simulink model "2025.1.21.methods"  (R2023a)
settings: Solver=ode4  StartTime=0.0  StopTime=40  FixedStep=dt  RelTol=1e-3
values from neighbouring files (symbols this model uses):
  AgN = Ag    [Copy_of_New_Ns.m]    (also in 旧数值子结构.m = zeros(ndof,1))
  C_phys_5dof = C    [旧静力凝聚.m]
  CNrt = CRrt    [Copy_of_New_Ns.m]    (also in 旧数值子结构.m)
  FN = zeros(15,1)    [Copy_of_New_Ns.m]    (also in 旧数值子结构.m = zeros(ndof,1))
  K_phys_5dof = K    [旧静力凝聚.m]
  KNbar_inv = inv(KNbar)    [Copy_of_New_Ns.m]    (also in 旧数值子结构.m)
  Koo = K(3:end,3:end)    [旧静力凝聚.m]
  Kot = K(3:end,1:2)    [旧静力凝聚.m]
  lN = l    [Copy_of_New_Ns.m]    (also in 旧数值子结构.m = zeros(ndof,1))
  M_phys_5dof = M    [旧静力凝聚.m]
  MNrt = diag([M1 1e-5 M6 M3 M2 M4 1e-5 M6 M3 M2 M1 M2 M3 M3 M2])    [Copy_of_New_Ns.m]    (also in 旧数值子结构.m = csvread("FE_Model/REF_SAP2000_Model/M_matrix.csv"))
  RNbar = zeros(15,1)    [Copy_of_New_Ns.m]    (also in 旧数值子结构.m = zeros(ndof,1))
undefined symbols (not defined in the file or in its folder): a0, a1, a2, a3, a4, a5, a6, a7, A_cplant, alpha1, alpha2, B_cplant, C_cplant, D_cplant, Dd_ss, delay, Ds_ss, dt, dv1, dv2, EQ_intensity, EQ_sw, Gnd_ss, Gns_ss, Hs1, Hs2, k3, k4, k6, K_lqr, KE, Mren, Muu, Phi_u2, Seed_snr
libraries: simulink x2, slpidlib x2, sldrtlib x1
(part 1 of 2)
settings Model: Creator=icu327  LastModifiedBy=liangyu
settings SolverCC: AlgebraicLoopSolver=TrustRegion
settings DataIOCC: SaveFormat=Array  ReturnWorkspaceOutputs=off
settings DebuggingCC: UnconnectedInputMsg=warning  UnconnectedOutputMsg=warning  UnconnectedLineMsg=warning  ArithmeticOperatorsInVariantConditions=warning
settings HardwareCC: ProdBitPerLong=64  ProdHWDeviceType=Intel->x86-64 (Linux 64)
settings ModelReferenceCC: EnableRefExpFcnMdlSchedulingChecks=on
settings SFSimCC: CustomCodeUndefinedFunction=UseInterfaceOnly
settings RTWCC: Description=Simulink Desktop Real-Time  SystemTargetFile=sldrt.tlc  TemplateMakefile=sldrt.tmf  RTWCompilerOptimization=on
settings CodeAppCC: MaxIdLength=95  StateflowObjectComments=on
settings SimulinkDesktopRealTimeCC: TargetLibSuffix=_sldrt.a  TargetPreCompLibLocation=C:\Program Files\MATLAB\R2023a\toolbox\sldrt\lib\win64

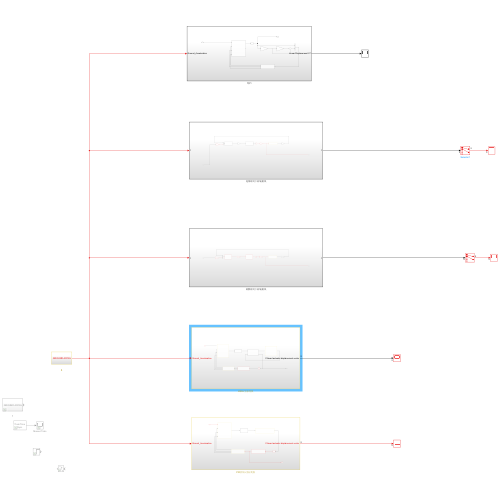
[thumbnail: Simulink's stored preview of the top-level diagram]
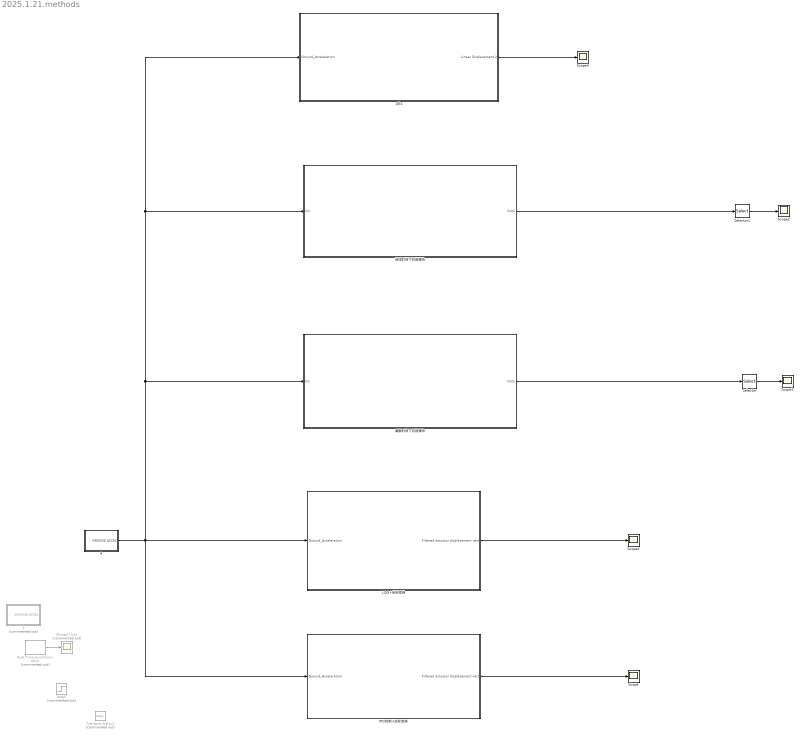
== system 2025.1.21.methods ==
  " 1" : Subsystem  Commented=on
  " 4" : Subsystem
  1阶1 : Subsystem
  LQG+坐标变换 : Subsystem
  Missed Ticks : Scope  Commented=on
  PID控制+坐标变换 : Subsystem
  Real-Time Synchronization : sldrtlib/Real-Time Synchronization  Commented=on  SampleTime=dt  MaxMissedTicks=10000  ShowMissedTicks=on  YieldWhenWaiting=off
  Scope{,1..4} (5 alike) : Scope
  Selector : Selector  InputPortWidth=5  IndexOptions=Index vector (dialog)  Indices=[1 2]  OutputSizes=1
  Selector1 : Selector  InputPortWidth=5  IndexOptions=Index vector (dialog)  Indices=[1 2]  OutputSizes=1
  Step5 : Step  Commented=on  SampleTime=0
  Transport Delay2 : TransportDelay  Commented=on  DelayTime=0.03
  离散时间下封装模块 : Subsystem
  连续时间下封装模块 : Subsystem
  wires:
  Real-Time Synchronization/1 -> Missed Ticks/1
  PID控制+坐标变换/1(Filtered actuator displacement vector) -> Scope/1
  LQG+坐标变换/1(Filtered actuator displacement vector) -> Scope3/1
  Selector/1 -> Scope1/1
  " 4"/1(GROUND ACCEL) -> PID控制+坐标变换/1(Ground_Acceleration), 离散时间下封装模块/1(In1), 1阶1/1(Ground_Acceleration), 连续时间下封装模块/1(In1), LQG+坐标变换/1(Ground_Acceleration)
  Selector1/1 -> Scope2/1
  连续时间下封装模块/1(Out1) -> Selector1/1
  离散时间下封装模块/1(Out1) -> Selector/1
  1阶1/1(Linear Displacement 27) -> Scope4/1

== system 2025.1.21.methods/ 1 ==
  note: Benchmark Control Problem for
      | Multi-axial Real-time Hybrid Simulation
      | Ground Acceleration
  Clock : Clock
  EQ scaling factor : Gain  Gain=EQ_intensity  Multiplication=Matrix(K*u)
  GROUND ACCELERATION : ToWorkspace  VariableName=EQ_input  SampleTime=-1
      settings: Save2DSignal=2-D array (concatenate along first dimension)
  Ground motion record : Subsystem
  Multiport Switch : MultiPortSwitch  SaturateOnIntegerOverflow=off  InputSameDT=off
  SWITCH CONSTANT : Constant  Value=EQ_sw
  To Workspace : ToWorkspace  VariableName=t  SampleTime=dt
  GROUND ACCEL : Outport  VectorParamsAs1DForOutWhenUnconnected=off
  wires:
  Multiport Switch/1 -> EQ scaling factor/1
  EQ scaling factor/1 -> GROUND ACCELERATION/1, GROUND ACCEL/1
  Ground motion record/1(El Centro) -> Multiport Switch/2
  Ground motion record/2(Kobe) -> Multiport Switch/3
  Ground motion record/3(Morgan) -> Multiport Switch/4
  SWITCH CONSTANT/1 -> Multiport Switch/1
  Clock/1 -> To Workspace/1

== system 2025.1.21.methods/ 4 ==
  note: Benchmark Control Problem for
      | Multi-axial Real-time Hybrid Simulation
      | Ground Acceleration
  Clock : Clock
  EQ scaling factor : Gain  Gain=EQ_intensity  Multiplication=Matrix(K*u)
  GROUND ACCELERATION : ToWorkspace  VariableName=EQ_input  SampleTime=-1
      settings: Save2DSignal=2-D array (concatenate along first dimension)
  Ground motion record : Subsystem
  Multiport Switch : MultiPortSwitch  SaturateOnIntegerOverflow=off  InputSameDT=off
  SWITCH CONSTANT : Constant  Value=EQ_sw
  To Workspace : ToWorkspace  VariableName=t  SampleTime=dt
  GROUND ACCEL : Outport  VectorParamsAs1DForOutWhenUnconnected=off
  wires:
  Multiport Switch/1 -> EQ scaling factor/1
  EQ scaling factor/1 -> GROUND ACCELERATION/1, GROUND ACCEL/1
  Ground motion record/1(El Centro) -> Multiport Switch/2
  Ground motion record/2(Kobe) -> Multiport Switch/3
  Ground motion record/3(Morgan) -> Multiport Switch/4
  SWITCH CONSTANT/1 -> Multiport Switch/1
  Clock/1 -> To Workspace/1

== system 2025.1.21.methods/1阶1 ==
  Ground_Acceleration : Inport
  " 数值子结构2" : Subsystem
      mask Display: image('$imagefile'); % Use "Edit Image" on toolstrip to change.
  Delay1 : Delay  DelayLength=delay
  Feedback Force Computation1 : Subsystem
  Mux : Mux  Inputs=2
  Sum : Sum  Inputs=|++
  动态位移 : Gain  Gain=Phi_u2*Phi_u2' * Muu  Multiplication=Matrix(K*u) (u vector)
  静态位移 : Gain  Gain=-Kuu \ Kuc  Multiplication=Matrix(K*u) (u vector)
  Linear Displacement 27 : Outport
  wires:
  动态位移/1 -> Sum/1
  " 数值子结构2"/1(Linear Displacement 27) -> Delay1/1
  Feedback Force Computation1/3(M(29)_phys (N*m)) -> " 数值子结构2"/4(RTHS_feedback_Moment29)  "Moment at Uncontrolled Node"
  静态位移/1 -> 动态位移/1, Sum/2
  Sum/1 -> Mux/2
  Feedback Force Computation1/2(M(21)_phys (N*m)) -> " 数值子结构2"/3(RTHS_feedback_Moment21)  "Moment at Controlled Node"
  Mux/1 -> Feedback Force Computation1/1("[x_est, theta_est] (m,rad)")
  Feedback Force Computation1/1(F(27)_phys (N)) -> " 数值子结构2"/2(RTHS_feedback_Force27)  "Feedback Force at Controlled Node"
  Ground_Acceleration/1 -> " 数值子结构2"/1(Ground_Acceleration)
  Delay1/1 -> Linear Displacement 27/1, 静态位移/1, Mux/1

== system 2025.1.21.methods/LQG+坐标变换 ==
  Ground_Acceleration : Inport
  " NUMERICAL SUBSTRUCTURE" : Subsystem
      mask Display: image('$imagefile'); % Use "Edit Image" on toolstrip to change.
  CONTROL PLANT : Subsystem
      mask Display: image('$imagefile'); % Use "Edit Image" on toolstrip to change.
  Coordinate transformation: Actuator to Frame : Subsystem
  Coordinate transformation: Frame to Actuator : Subsystem
  Delay3 : Delay  DelayLength=delay
  Feedback Force Computation3 : Subsystem
  MIMO CONTROLLER : Subsystem
  Filtered actuator displacement vector : Outport
  wires:
  Feedback Force Computation3/1(F(27)_phys (N)) -> " NUMERICAL SUBSTRUCTURE"/2(RTHS_feedback_Force27)  "Feedback Force at Controlled Node"
  CONTROL PLANT/1(Out1) -> MIMO CONTROLLER/2("[xm1, xm2] (mm)")  "Measured actuator displacement vector (mm)"
  MIMO CONTROLLER/1("[u1, u2] (mm)") -> CONTROL PLANT/1(In1)  "Command input vector Actuator coordinates"
  Coordinate transformation: Frame to Actuator/1("[xa1,xa2] mm") -> MIMO CONTROLLER/1("[xa1, xa2] (mm)")  "Target actuator displacement vector (mm)"
  MIMO CONTROLLER/2("[xm1_est, xm2_est] (mm)") -> Filtered actuator displacement vector/1, Delay3/1  "Filtered actuator displacement vector"
  Feedback Force Computation3/3(M(29)_phys (N*m)) -> " NUMERICAL SUBSTRUCTURE"/4(RTHS_feedback_Moment29)  "Moment at Uncontrolled Node"
  Ground_Acceleration/1 -> " NUMERICAL SUBSTRUCTURE"/1(Ground_Acceleration)
  " NUMERICAL SUBSTRUCTURE"/1(Linear Displacement 27) -> Coordinate transformation: Frame to Actuator/1("[x, theta]")  "Target displacement vector Frame coordinates (mm, rad)"
  Coordinate transformation: Actuator to Frame/1("[x, theta] (m, rad)") -> Feedback Force Computation3/1("[x_est, theta_est] (m,rad)")
  Feedback Force Computation3/2(M(21)_phys (N*m)) -> " NUMERICAL SUBSTRUCTURE"/3(RTHS_feedback_Moment21)  "Moment at Controlled Node"
  Delay3/1 -> Coordinate transformation: Actuator to Frame/1("[xm1_est, xm2_est] (mm)")

== system 2025.1.21.methods/PID控制+坐标变换 ==
  Ground_Acceleration : Inport
  " 数值子结构" : Subsystem
      mask Display: image('$imagefile'); % Use "Edit Image" on toolstrip to change.
  Delay : Delay  DelayLength=delay
  Feedback Force Computation : Subsystem
  "坐标转换 此处将两个作动器的位移转为 横向位移与节点转角 " : Subsystem
  坐标转换 此处将横向位移与节点转角转为 两个作动器的位移 : Subsystem
  控制器与作动器 : Subsystem
  Filtered actuator displacement vector : Outport
  wires:
  Feedback Force Computation/1(F(27)_phys (N)) -> " 数值子结构"/2(RTHS_feedback_Force27)  "Feedback Force at Controlled Node"
  坐标转换 此处将横向位移与节点转角转为 两个作动器的位移/1("[xa1,xa2] mm") -> 控制器与作动器/1(Target actuator displacement vector (mm))  "Target actuator displacement vector (mm)"
  Feedback Force Computation/2(M(21)_phys (N*m)) -> " 数值子结构"/3(RTHS_feedback_Moment21)  "Moment at Controlled Node"
  控制器与作动器/1(Filtered actuator displacement vector) -> Delay/1
  "坐标转换 此处将两个作动器的位移转为 横向位移与节点转角 "/1("[x, theta] (m, rad)") -> Filtered actuator displacement vector/1, Feedback Force Computation/1("[x_est, theta_est] (m,rad)")
  " 数值子结构"/1(Linear Displacement 27) -> 坐标转换 此处将横向位移与节点转角转为 两个作动器的位移/1("[x, theta]")  "Target displacement vector Frame coordinates (mm, rad)"
  Ground_Acceleration/1 -> " 数值子结构"/1(Ground_Acceleration)
  Feedback Force Computation/3(M(29)_phys (N*m)) -> " 数值子结构"/4(RTHS_feedback_Moment29)  "Moment at Uncontrolled Node"
  Delay/1 -> "坐标转换 此处将两个作动器的位移转为 横向位移与节点转角 "/1("[xm1_est, xm2_est] (mm)")

== system 2025.1.21.methods/离散时间下封装模块 ==
  In1 : Inport
  Delay : Delay  DelayLength=delay
  Discrete State-Space : DiscreteStateSpace  A=Gnd_ss.A  B=Gnd_ss.B  C=Gnd_ss.C  D=Gnd_ss.D  SampleTime=1/1024
  Feedback Force Computation2 : Subsystem
  Gain5 : Gain  Gain=k3  Multiplication=Matrix(K*u)
  PID : DiscreteStateSpace  A=Dd_ss.A  B=Dd_ss.B  C=Dd_ss.C  D=Dd_ss.D  SampleTime=1/1024
  Sum1 : Sum  Inputs=-|+
  坐标转换 : Gain  Gain=Hs1*k6*1e3  Multiplication=Matrix(K*u)
  坐标转换2 : Gain  Gain=k4*Hs2*1e-3  Multiplication=Matrix(K*u)
  将加速度转为力 : Gain  Gain=-Mren*[1;0;1;1;0]  Multiplication=Matrix(K*u)
  Out1 : Outport
  wires:
  Feedback Force Computation2/1(F(27)_phys (N)) -> Gain5/1
  坐标转换/1 -> PID/1
  Delay/1 -> 坐标转换2/1
  Gain5/1 -> Sum1/1
  PID/1 -> Delay/1
  将加速度转为力/1 -> Sum1/2
  In1/1 -> 将加速度转为力/1
  Sum1/1 -> Discrete State-Space/1
  坐标转换2/1 -> Out1/1, Feedback Force Computation2/1("[x_est, theta_est] (m,rad)")
  Discrete State-Space/1 -> 坐标转换/1  "state版"

== system 2025.1.21.methods/连续时间下封装模块 ==
  In1 : Inport
  Delay1 : Delay  DelayLength=delay
  Feedback Force Computation1 : Subsystem
  Gain1 : Gain  Gain=k3  Multiplication=Matrix(K*u)
  PID : StateSpace  A=Ds_ss.A  B=Ds_ss.B  C=Ds_ss.C  D=Ds_ss.D  InitialCondition=0
  Sum2 : Sum  Inputs=-|+
  坐标转换1 : Gain  Gain=Hs1*k6*1e3  Multiplication=Matrix(K*u)
  坐标转换3 : Gain  Gain=k4*Hs2*1e-3  Multiplication=Matrix(K*u)
  将加速度转为力1 : Gain  Gain=-Mren*[1;0;1;1;0]  Multiplication=Matrix(K*u)
  连续数值子结构 : StateSpace  A=Gns_ss.A  B=Gns_ss.B  C=Gns_ss.C  D=Gns_ss.D  InitialCondition=0
  Out1 : Outport
  wires:
  Feedback Force Computation1/1(F(27)_phys (N)) -> Gain1/1
  Gain1/1 -> Sum2/1
  Delay1/1 -> 坐标转换3/1
  连续数值子结构/1 -> 坐标转换1/1  "state版"
  PID/1 -> Delay1/1
  坐标转换3/1 -> Out1/1, Feedback Force Computation1/1("[x_est, theta_est] (m,rad)")
  坐标转换1/1 -> PID/1
  将加速度转为力1/1 -> Sum2/2
  Sum2/1 -> 连续数值子结构/1
  In1/1 -> 将加速度转为力1/1

== system 2025.1.21.methods/ 1/Ground motion record ==
  From File : FromFile  FileName=ElCentroAccelNoScaling.mat  SampleTime=dt
  From File1 : FromFile  FileName=KobeAccelNoScaling.mat  SampleTime=dt
  From File2 : FromFile  FileName=MorganAccelNoScaling.mat  SampleTime=dt
  El Centro : Outport
  Kobe : Outport  Port=2
  Morgan : Outport  Port=3
  wires:
  From File/1 -> El Centro/1
  From File2/1 -> Morgan/1
  From File1/1 -> Kobe/1

== system 2025.1.21.methods/ 4/Ground motion record ==
  From File : FromFile  FileName=D:\matlab\LY\gitee\liangyustability\simulink模型修改\Ground_motions\ElCentroAccelNoScaling.mat  SampleTime=dt
  From File1 : FromFile  FileName=D:\matlab\LY\gitee\liangyustability\simulink模型修改\Ground_motions\KobeAccelNoScaling.mat  SampleTime=dt
  From File2 : FromFile  FileName=D:\matlab\LY\gitee\liangyustability\simulink模型修改\Ground_motions\MorganAccelNoScaling.mat  SampleTime=dt
  El Centro : Outport
  Kobe : Outport  Port=2
  Morgan : Outport  Port=3
  wires:
  From File/1 -> El Centro/1
  From File2/1 -> Morgan/1
  From File1/1 -> Kobe/1

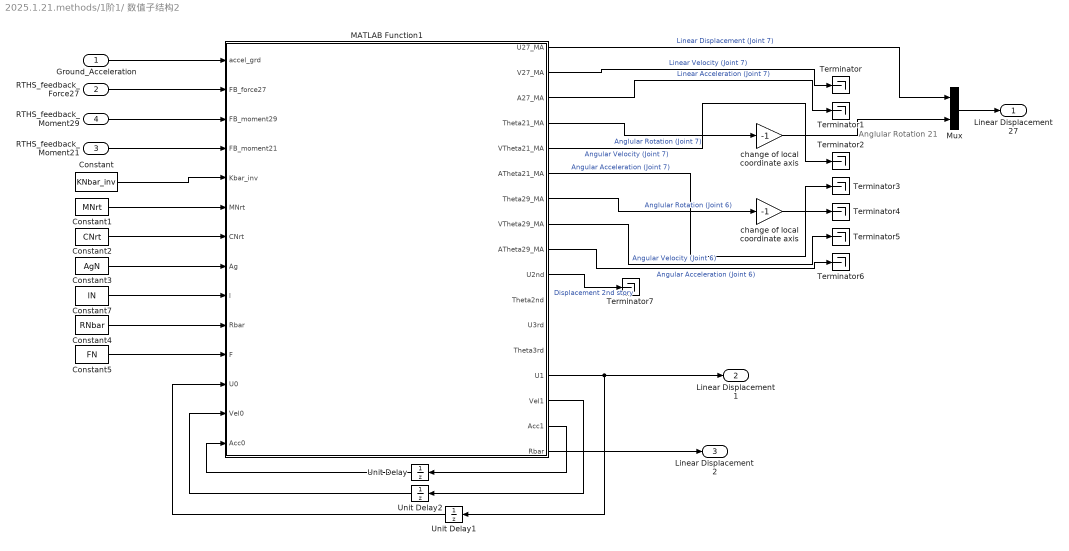
== system 2025.1.21.methods/1阶1/ 数值子结构2 ==
  note: Anglular Rotation 21
  Ground_Acceleration : Inport
  RTHS_feedback_Force27 : Inport  Port=2
  RTHS_feedback_Moment21 : Inport  Port=3
  RTHS_feedback_Moment29 : Inport  Port=4
  Constant : Constant  Value=KNbar_inv  VectorParams1D=off
  Constant1 : Constant  Value=MNrt  VectorParams1D=off
  Constant2 : Constant  Value=CNrt  VectorParams1D=off
  Constant3 : Constant  Value=AgN  VectorParams1D=off
  Constant4 : Constant  Value=RNbar  VectorParams1D=off
  Constant5 : Constant  Value=FN  VectorParams1D=off
  Constant7 : Constant  Value=lN  VectorParams1D=off
  MATLAB Function1 : MATLAB Function  TreatAsAtomicUnit=on
  Mux : Mux  Inputs=2
  Terminator{,1..7} (8 alike) : Terminator
  Unit Delay : UnitDelay  SampleTime=-1  HasFrameUpgradeWarning=on
  Unit Delay1 : UnitDelay  SampleTime=-1  HasFrameUpgradeWarning=on
  Unit Delay2 : UnitDelay  SampleTime=-1  HasFrameUpgradeWarning=on
  change of local coordinate axis : Gain  Gain=-1
  "change of local coordinate axis  " : Gain  Gain=-1
  Linear Displacement 27 : Outport  VectorParamsAs1DForOutWhenUnconnected=off
  Linear Displacement 1 : Outport  Port=2  VectorParamsAs1DForOutWhenUnconnected=off
  Linear Displacement 2 : Outport  Port=3  VectorParamsAs1DForOutWhenUnconnected=off
  wires:
  Ground_Acceleration/1 -> MATLAB Function1/1(accel_grd)
  RTHS_feedback_Force27/1 -> MATLAB Function1/2(FB_force27)
  RTHS_feedback_Moment29/1 -> MATLAB Function1/3(FB_moment29)
  MATLAB Function1/1(U27_MA) -> Mux/1  "Linear Displacement (Joint 7)"
  MATLAB Function1/4(Theta21_MA) -> change of local coordinate axis/1  "Anglular Rotation (Joint 7)"
  Constant/1 -> MATLAB Function1/5(Kbar_inv)
  Constant1/1 -> MATLAB Function1/6(MNrt)
  Constant2/1 -> MATLAB Function1/7(CNrt)
  Constant3/1 -> MATLAB Function1/8(Ag)
  Constant7/1 -> MATLAB Function1/9(l)
  Constant4/1 -> MATLAB Function1/10("Rbar ")
  Unit Delay1/1 -> MATLAB Function1/12(U0)
  Unit Delay2/1 -> MATLAB Function1/13(Vel0)
  Unit Delay/1 -> MATLAB Function1/14(Acc0)
  MATLAB Function1/15(Vel1) -> Unit Delay2/1
  MATLAB Function1/16(Acc1) -> Unit Delay/1
  Constant5/1 -> MATLAB Function1/11(F)
  MATLAB Function1/2(V27_MA) -> Terminator/1  "Linear Velocity (Joint 7)"
  MATLAB Function1/3(A27_MA) -> Terminator1/1  "Linear Acceleration (Joint 7)"
  MATLAB Function1/5(VTheta21_MA) -> Terminator2/1  "Angular Velocity (Joint 7)"
  MATLAB Function1/6(ATheta21_MA) -> Terminator3/1  "Angular Acceleration (Joint 7)"
  MATLAB Function1/9(ATheta29_MA) -> Terminator6/1  "Angular Acceleration (Joint 6)"
  MATLAB Function1/8(VTheta29_MA) -> Terminator5/1  "Angular Velocity (Joint 6)"
  MATLAB Function1/7(Theta29_MA) -> "change of local coordinate axis  "/1  "Anglular Rotation (Joint 6)"
  RTHS_feedback_Moment21/1 -> MATLAB Function1/4(FB_moment21)
  change of local coordinate axis/1 -> Mux/2
  "change of local coordinate axis  "/1 -> Terminator4/1
  Mux/1 -> Linear Displacement 27/1
  MATLAB Function1/10(U2nd) -> Terminator7/1  "Displacement 2nd story"
  MATLAB Function1/14(U1) -> Unit Delay1/1, Linear Displacement 1/1
  MATLAB Function1/17(Rbar) -> Linear Displacement 2/1

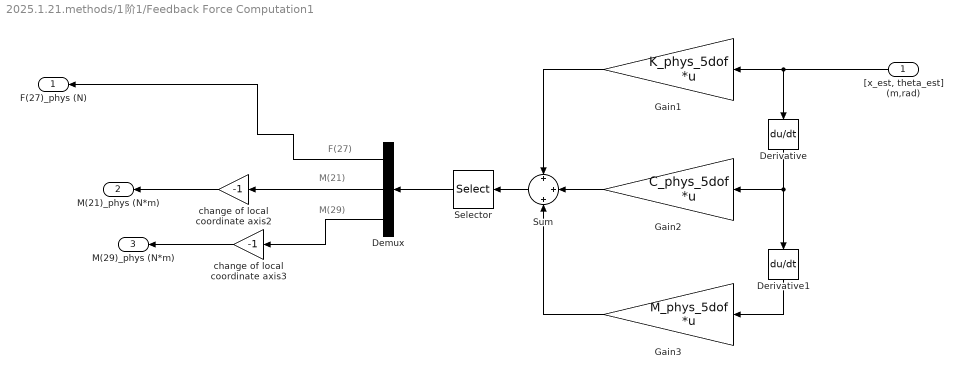
== system 2025.1.21.methods/1阶1/Feedback Force Computation1 ==
  note: F(27)
  note: M(21)
  note: M(29)
  "[x_est, theta_est] (m,rad)" : Inport
  Demux : Demux  Outputs=3
  Derivative : Derivative
  Derivative1 : Derivative
  Gain1 : Gain  Gain=K_phys_5dof  Multiplication=Matrix(K*u) (u vector)
  Gain2 : Gain  Gain=C_phys_5dof  Multiplication=Matrix(K*u) (u vector)
  Gain3 : Gain  Gain=M_phys_5dof  Multiplication=Matrix(K*u) (u vector)
  Selector : Selector  InputPortWidth=5  IndexOptions=Index vector (dialog)  Indices=[1 2 3]  OutputSizes=1
  Sum : Sum  Inputs=+|+|+
  change of local coordinate axis2 : Gain  Gain=-1
  change of local coordinate axis3 : Gain  Gain=-1
  F(27)_phys (N) : Outport  VectorParamsAs1DForOutWhenUnconnected=off
  M(21)_phys (N*m) : Outport  Port=2  VectorParamsAs1DForOutWhenUnconnected=off
  M(29)_phys (N*m) : Outport  Port=3  VectorParamsAs1DForOutWhenUnconnected=off
  wires:
  Derivative1/1 -> Gain3/1
  Gain2/1 -> Sum/2
  Derivative/1 -> Gain2/1, Derivative1/1
  Gain1/1 -> Sum/1
  Demux/1 -> F(27)_phys (N)/1
  Sum/1 -> Selector/1
  Selector/1 -> Demux/1
  Gain3/1 -> Sum/3
  Demux/2 -> change of local coordinate axis2/1
  Demux/3 -> change of local coordinate axis3/1
  "[x_est, theta_est] (m,rad)"/1 -> Derivative/1, Gain1/1
  change of local coordinate axis2/1 -> M(21)_phys (N*m)/1
  change of local coordinate axis3/1 -> M(29)_phys (N*m)/1

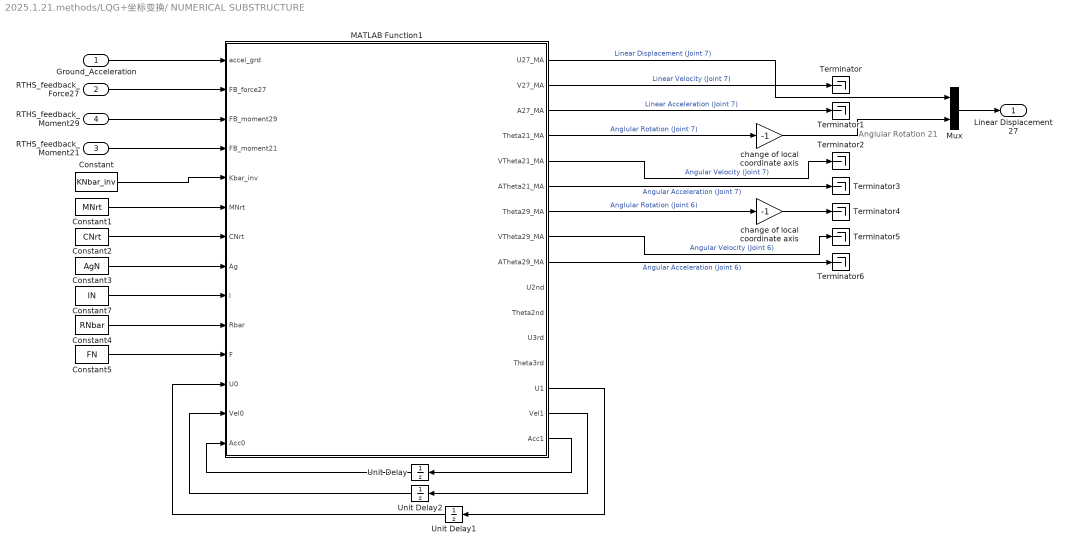
== system 2025.1.21.methods/LQG+坐标变换/ NUMERICAL SUBSTRUCTURE ==
  note: Anglular Rotation 21
  Ground_Acceleration : Inport
  RTHS_feedback_Force27 : Inport  Port=2
  RTHS_feedback_Moment21 : Inport  Port=3
  RTHS_feedback_Moment29 : Inport  Port=4
  Constant : Constant  Value=KNbar_inv  VectorParams1D=off
  Constant1 : Constant  Value=MNrt  VectorParams1D=off
  Constant2 : Constant  Value=CNrt  VectorParams1D=off
  Constant3 : Constant  Value=AgN  VectorParams1D=off
  Constant4 : Constant  Value=RNbar  VectorParams1D=off
  Constant5 : Constant  Value=FN  VectorParams1D=off
  Constant7 : Constant  Value=lN  VectorParams1D=off
  MATLAB Function1 : MATLAB Function  TreatAsAtomicUnit=on
  Mux : Mux  Inputs=2
  Terminator{,1..6} (7 alike) : Terminator
  Unit Delay : UnitDelay  SampleTime=-1  HasFrameUpgradeWarning=on
  Unit Delay1 : UnitDelay  SampleTime=-1  HasFrameUpgradeWarning=on
  Unit Delay2 : UnitDelay  SampleTime=-1  HasFrameUpgradeWarning=on
  change of local coordinate axis : Gain  Gain=-1
  "change of local coordinate axis  " : Gain  Gain=-1
  Linear Displacement 27 : Outport  VectorParamsAs1DForOutWhenUnconnected=off
  wires:
  Ground_Acceleration/1 -> MATLAB Function1/1(accel_grd)
  RTHS_feedback_Force27/1 -> MATLAB Function1/2(FB_force27)
  RTHS_feedback_Moment29/1 -> MATLAB Function1/3(FB_moment29)
  MATLAB Function1/1(U27_MA) -> Mux/1  "Linear Displacement (Joint 7)"
  MATLAB Function1/4(Theta21_MA) -> change of local coordinate axis/1  "Anglular Rotation (Joint 7)"
  Constant/1 -> MATLAB Function1/5(Kbar_inv)
  Constant1/1 -> MATLAB Function1/6(MNrt)
  Constant2/1 -> MATLAB Function1/7(CNrt)
  Constant3/1 -> MATLAB Function1/8(Ag)
  Constant7/1 -> MATLAB Function1/9(l)
  Constant4/1 -> MATLAB Function1/10(Rbar)
  Unit Delay1/1 -> MATLAB Function1/12(U0)
  Unit Delay2/1 -> MATLAB Function1/13(Vel0)
  Unit Delay/1 -> MATLAB Function1/14(Acc0)
  MATLAB Function1/15(Vel1) -> Unit Delay2/1
  MATLAB Function1/16(Acc1) -> Unit Delay/1
  MATLAB Function1/14(U1) -> Unit Delay1/1
  Constant5/1 -> MATLAB Function1/11(F)
  MATLAB Function1/2(V27_MA) -> Terminator/1  "Linear Velocity (Joint 7)"
  MATLAB Function1/3(A27_MA) -> Terminator1/1  "Linear Acceleration (Joint 7)"
  MATLAB Function1/5(VTheta21_MA) -> Terminator2/1  "Angular Velocity (Joint 7)"
  MATLAB Function1/6(ATheta21_MA) -> Terminator3/1  "Angular Acceleration (Joint 7)"
  MATLAB Function1/9(ATheta29_MA) -> Terminator6/1  "Angular Acceleration (Joint 6)"
  MATLAB Function1/8(VTheta29_MA) -> Terminator5/1  "Angular Velocity (Joint 6)"
  MATLAB Function1/7(Theta29_MA) -> "change of local coordinate axis  "/1  "Anglular Rotation (Joint 6)"
  RTHS_feedback_Moment21/1 -> MATLAB Function1/4(FB_moment21)
  change of local coordinate axis/1 -> Mux/2
  "change of local coordinate axis  "/1 -> Terminator4/1
  Mux/1 -> Linear Displacement 27/1

== system 2025.1.21.methods/LQG+坐标变换/CONTROL PLANT ==
  In1 : Inport
  Control Plant : StateSpace  A=A_cplant  B=B_cplant  C=C_cplant  D=D_cplant  InitialCondition=0
  Demux : Demux  Outputs=2
  Mux : Mux  Inputs=2
  Sensor Noise 3 : simulink/Sources/Band-Limited White Noise  Cov=rms_noise_DT  Ts=dt  seed=double(Seed_snr.Seed)
  Sensor Noise 4 : simulink/Sources/Band-Limited White Noise  Cov=rms_noise_DT  Ts=dt  seed=double(Seed_snr.Seed)
  Sum : Sum  Inputs=++|
  Sum1 : Sum  Inputs=|++
  Out1 : Outport
  wires:
  Control Plant/1 -> Demux/1
  In1/1 -> Control Plant/1
  Demux/2 -> Sum1/1
  Demux/1 -> Sum/2
  Mux/1 -> Out1/1  "[u1,u2] (mm)"
  Sensor Noise 3/1 -> Sum/1
  Sensor Noise 4/1 -> Sum1/2
  Sum/1 -> Mux/1
  Sum1/1 -> Mux/2

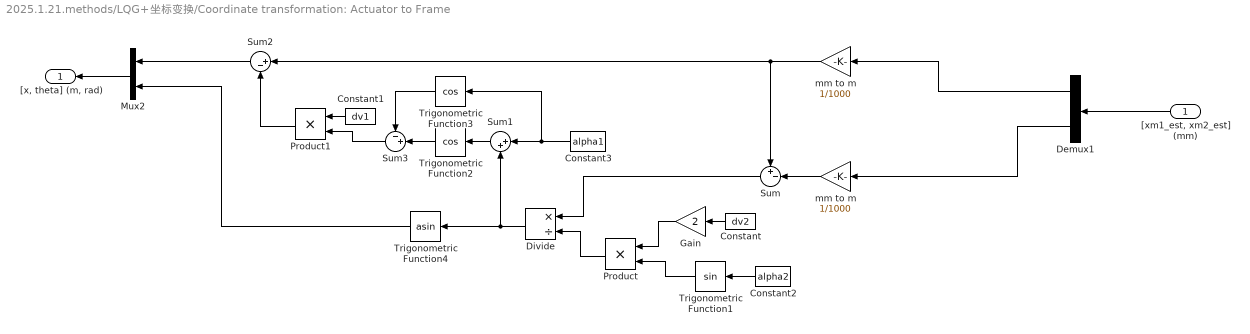
== system 2025.1.21.methods/LQG+坐标变换/Coordinate transformation: Actuator to Frame ==
  "[xm1_est, xm2_est] (mm)" : Inport
  Constant : Constant  Value=dv2
  Constant1 : Constant  Value=dv1
  Constant2 : Constant  Value=alpha2
  Constant3 : Constant  Value=alpha1
  Demux1 : Demux  Outputs=2
  Divide : Product  Inputs=*/
  Gain : Gain  Gain=2
  Mux2 : Mux  Inputs=2
  Product : Product
  Product1 : Product
  Sum : Sum  Inputs=+-|
  Sum1 : Sum  Inputs=|++
  Sum2 : Sum  Inputs=|+-
  Sum3 : Sum  Inputs=-+|
  Trigonometric Function1 : Trigonometry
  Trigonometric Function2 : Trigonometry  Operator=cos
  Trigonometric Function3 : Trigonometry  Operator=cos
  Trigonometric Function4 : Trigonometry  Operator=asin
  mm to m : Gain  Gain=1/1000
  "mm to m " : Gain  Gain=1/1000
  "[x, theta] (m, rad)" : Outport  VectorParamsAs1DForOutWhenUnconnected=off
  wires:
  Constant2/1 -> Trigonometric Function1/1
  Constant1/1 -> Product1/1
  Demux1/1 -> mm to m/1
  Demux1/2 -> "mm to m "/1
  Sum/1 -> Divide/1
  Constant/1 -> Gain/1
  Trigonometric Function1/1 -> Product/2
  Gain/1 -> Product/1
  Product/1 -> Divide/2
  Divide/1 -> Sum1/2, Trigonometric Function4/1
  Sum1/1 -> Trigonometric Function2/1
  Constant3/1 -> Sum1/1, Trigonometric Function3/1
  Sum3/1 -> Product1/2
  Sum2/1 -> Mux2/1
  Trigonometric Function2/1 -> Sum3/2
  Trigonometric Function3/1 -> Sum3/1
  Product1/1 -> Sum2/2
  mm to m/1 -> Sum2/1, Sum/1
  "mm to m "/1 -> Sum/2
  Trigonometric Function4/1 -> Mux2/2
  "[xm1_est, xm2_est] (mm)"/1 -> Demux1/1
  Mux2/1 -> "[x, theta] (m, rad)"/1

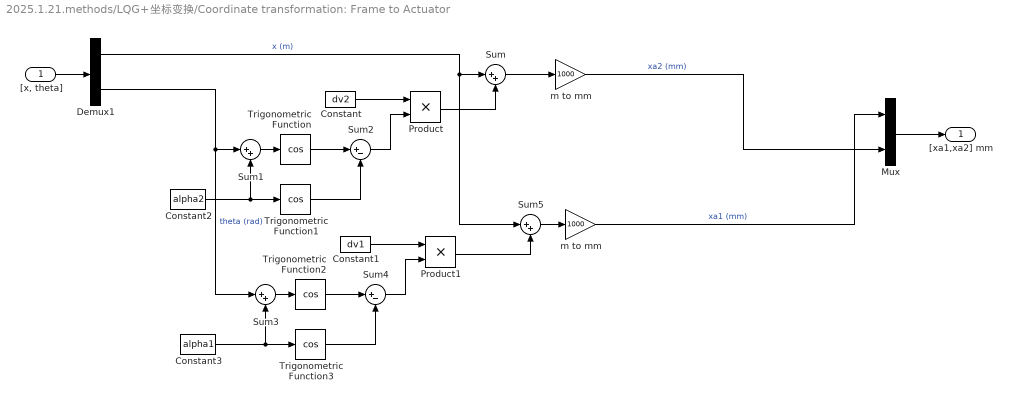
== system 2025.1.21.methods/LQG+坐标变换/Coordinate transformation: Frame to Actuator ==
  "[x, theta]" : Inport
  Constant : Constant  Value=dv2
  Constant1 : Constant  Value=dv1
  Constant2 : Constant  Value=alpha2
  Constant3 : Constant  Value=alpha1
  Demux1 : Demux  Outputs=2
  Mux : Mux  Inputs=2
  Product : Product
  Product1 : Product
  Sum{,1,3,5} (4 alike) : Sum  Inputs=|++
  Sum2 : Sum  Inputs=|+-
  Sum4 : Sum  Inputs=|+-
  Trigonometric Function{,1..3} (4 alike) : Trigonometry  Operator=cos
  m to mm : Gain  Gain=1000
  "m to mm " : Gain  Gain=1000
  "[xa1,xa2] mm" : Outport  VectorParamsAs1DForOutWhenUnconnected=off
  wires:
  Constant/1 -> Product/1
  Constant2/1 -> Sum1/2, Trigonometric Function1/1
  Sum1/1 -> Trigonometric Function/1
  Trigonometric Function/1 -> Sum2/1
  Trigonometric Function1/1 -> Sum2/2
  Sum2/1 -> Product/2
  Product/1 -> Sum/2
  Sum/1 -> m to mm/1
  Sum4/1 -> Product1/2
  Trigonometric Function3/1 -> Sum4/2
  Trigonometric Function2/1 -> Sum4/1
  Sum3/1 -> Trigonometric Function2/1
  Constant3/1 -> Sum3/2, Trigonometric Function3/1
  Constant1/1 -> Product1/1
  Product1/1 -> Sum5/2
  Sum5/1 -> "m to mm "/1
  "m to mm "/1 -> Mux/1  "xa1 (mm)"
  m to mm/1 -> Mux/2  "xa2 (mm)"
  Demux1/1 -> Sum/1, Sum5/1  "x (m)"
  "[x, theta]"/1 -> Demux1/1
  Demux1/2 -> Sum3/1, Sum1/1  "theta (rad)"
  Mux/1 -> "[xa1,xa2] mm"/1

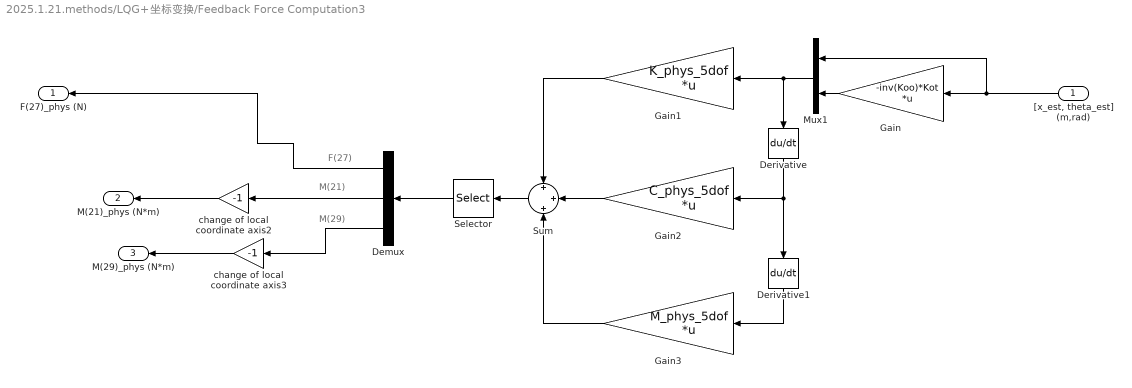
== system 2025.1.21.methods/LQG+坐标变换/Feedback Force Computation3 ==
  note: F(27)
  note: M(21)
  note: M(29)
  "[x_est, theta_est] (m,rad)" : Inport
  Demux : Demux  Outputs=3
  Derivative : Derivative
  Derivative1 : Derivative
  Gain : Gain  Gain=-inv(Koo)*Kot  Multiplication=Matrix(K*u) (u vector)
  Gain1 : Gain  Gain=K_phys_5dof  Multiplication=Matrix(K*u) (u vector)
  Gain2 : Gain  Gain=C_phys_5dof  Multiplication=Matrix(K*u) (u vector)
  Gain3 : Gain  Gain=M_phys_5dof  Multiplication=Matrix(K*u) (u vector)
  Mux1 : Mux  Inputs=2
  Selector : Selector  InputPortWidth=5  IndexOptions=Index vector (dialog)  Indices=[1 2 3]  OutputSizes=1
  Sum : Sum  Inputs=+|+|+
  change of local coordinate axis2 : Gain  Gain=-1
  change of local coordinate axis3 : Gain  Gain=-1
  F(27)_phys (N) : Outport  VectorParamsAs1DForOutWhenUnconnected=off
  M(21)_phys (N*m) : Outport  Port=2  VectorParamsAs1DForOutWhenUnconnected=off
  M(29)_phys (N*m) : Outport  Port=3  VectorParamsAs1DForOutWhenUnconnected=off
  wires:
  Gain/1 -> Mux1/2
  Derivative1/1 -> Gain3/1
  Gain2/1 -> Sum/2
  Derivative/1 -> Gain2/1, Derivative1/1
  Gain1/1 -> Sum/1
  "[x_est, theta_est] (m,rad)"/1 -> Gain/1, Mux1/1
  Demux/1 -> F(27)_phys (N)/1
  Sum/1 -> Selector/1
  Selector/1 -> Demux/1
  Gain3/1 -> Sum/3
  Demux/2 -> change of local coordinate axis2/1
  Demux/3 -> change of local coordinate axis3/1
  Mux1/1 -> Derivative/1, Gain1/1
  change of local coordinate axis2/1 -> M(21)_phys (N*m)/1
  change of local coordinate axis3/1 -> M(29)_phys (N*m)/1

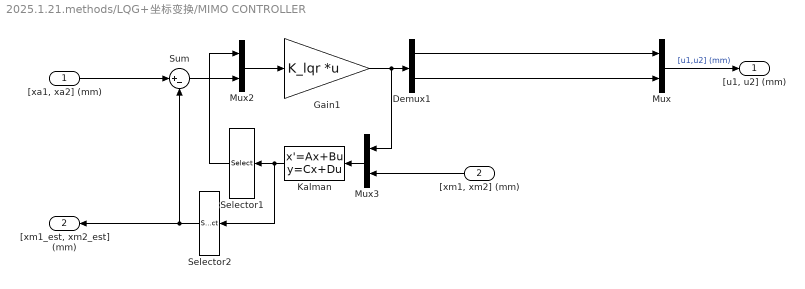
== system 2025.1.21.methods/LQG+坐标变换/MIMO CONTROLLER ==
  "[xa1, xa2] (mm)" : Inport
  "[xm1, xm2] (mm)" : Inport  Port=2
  Demux1 : Demux  Outputs=2
  Gain1 : Gain  Gain=K_lqr  Multiplication=Matrix(K*u) (u vector)
  Kalman : StateSpace  A=KE.A  B=KE.B  C=KE.C  D=KE.D  InitialCondition=0
  Mux : Mux  Inputs=2
  Mux2 : Mux  Inputs=2
  Mux3 : Mux  Inputs=2
  Selector1 : Selector  InputPortWidth=10  IndexOptions=Index vector (dialog)  Indices=[3:10]  OutputSizes=1
  Selector2 : Selector  InputPortWidth=10  IndexOptions=Index vector (dialog)  Indices=[1:2]  OutputSizes=1
  Sum : Sum  Inputs=|+-
  "[u1, u2] (mm)" : Outport  VectorParamsAs1DForOutWhenUnconnected=off
  "[xm1_est, xm2_est] (mm)" : Outport  Port=2  VectorParamsAs1DForOutWhenUnconnected=off
  wires:
  "[xa1, xa2] (mm)"/1 -> Sum/1
  Selector1/1 -> Mux2/1
  Kalman/1 -> Selector2/1, Selector1/1
  Mux3/1 -> Kalman/1
  Sum/1 -> Mux2/2
  Selector2/1 -> Sum/2, "[xm1_est, xm2_est] (mm)"/1
  Gain1/1 -> Mux3/1, Demux1/1
  Mux2/1 -> Gain1/1
  Demux1/1 -> Mux/1
  Demux1/2 -> Mux/2
  Mux/1 -> "[u1, u2] (mm)"/1  "[u1,u2] (mm)"
  "[xm1, xm2] (mm)"/1 -> Mux3/2

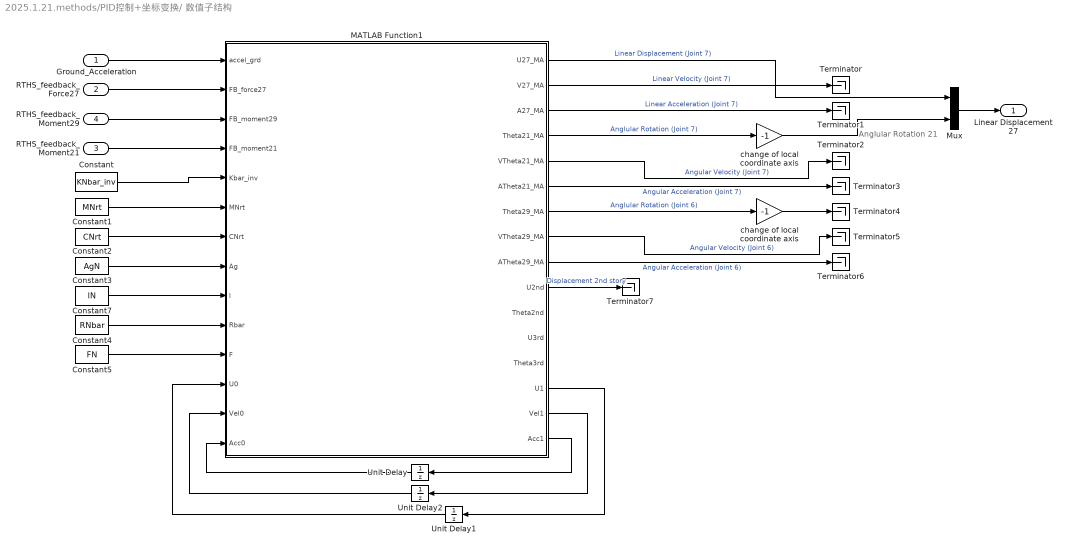
== system 2025.1.21.methods/PID控制+坐标变换/ 数值子结构 ==
  note: Anglular Rotation 21
  Ground_Acceleration : Inport
  RTHS_feedback_Force27 : Inport  Port=2
  RTHS_feedback_Moment21 : Inport  Port=3
  RTHS_feedback_Moment29 : Inport  Port=4
  Constant : Constant  Value=KNbar_inv  VectorParams1D=off
  Constant1 : Constant  Value=MNrt  VectorParams1D=off
  Constant2 : Constant  Value=CNrt  VectorParams1D=off
  Constant3 : Constant  Value=AgN  VectorParams1D=off
  Constant4 : Constant  Value=RNbar  VectorParams1D=off
  Constant5 : Constant  Value=FN  VectorParams1D=off
  Constant7 : Constant  Value=lN  VectorParams1D=off
  MATLAB Function1 : MATLAB Function  TreatAsAtomicUnit=on
  Mux : Mux  Inputs=2
  Terminator{,1..7} (8 alike) : Terminator
  Unit Delay : UnitDelay  SampleTime=-1  HasFrameUpgradeWarning=on
  Unit Delay1 : UnitDelay  SampleTime=-1  HasFrameUpgradeWarning=on
  Unit Delay2 : UnitDelay  SampleTime=-1  HasFrameUpgradeWarning=on
  change of local coordinate axis : Gain  Gain=-1
  "change of local coordinate axis  " : Gain  Gain=-1
  Linear Displacement 27 : Outport  VectorParamsAs1DForOutWhenUnconnected=off
  wires:
  Ground_Acceleration/1 -> MATLAB Function1/1(accel_grd)
  RTHS_feedback_Force27/1 -> MATLAB Function1/2(FB_force27)
  RTHS_feedback_Moment29/1 -> MATLAB Function1/3(FB_moment29)
  MATLAB Function1/1(U27_MA) -> Mux/1  "Linear Displacement (Joint 7)"
  MATLAB Function1/4(Theta21_MA) -> change of local coordinate axis/1  "Anglular Rotation (Joint 7)"
  Constant/1 -> MATLAB Function1/5(Kbar_inv)
  Constant1/1 -> MATLAB Function1/6(MNrt)
  Constant2/1 -> MATLAB Function1/7(CNrt)
  Constant3/1 -> MATLAB Function1/8(Ag)
  Constant7/1 -> MATLAB Function1/9(l)
  Constant4/1 -> MATLAB Function1/10(Rbar)
  Unit Delay1/1 -> MATLAB Function1/12(U0)
  Unit Delay2/1 -> MATLAB Function1/13(Vel0)
  Unit Delay/1 -> MATLAB Function1/14(Acc0)
  MATLAB Function1/15(Vel1) -> Unit Delay2/1
  MATLAB Function1/16(Acc1) -> Unit Delay/1
  MATLAB Function1/14(U1) -> Unit Delay1/1
  Constant5/1 -> MATLAB Function1/11(F)
  MATLAB Function1/2(V27_MA) -> Terminator/1  "Linear Velocity (Joint 7)"
  MATLAB Function1/3(A27_MA) -> Terminator1/1  "Linear Acceleration (Joint 7)"
  MATLAB Function1/5(VTheta21_MA) -> Terminator2/1  "Angular Velocity (Joint 7)"
  MATLAB Function1/6(ATheta21_MA) -> Terminator3/1  "Angular Acceleration (Joint 7)"
  MATLAB Function1/9(ATheta29_MA) -> Terminator6/1  "Angular Acceleration (Joint 6)"
  MATLAB Function1/8(VTheta29_MA) -> Terminator5/1  "Angular Velocity (Joint 6)"
  MATLAB Function1/7(Theta29_MA) -> "change of local coordinate axis  "/1  "Anglular Rotation (Joint 6)"
  RTHS_feedback_Moment21/1 -> MATLAB Function1/4(FB_moment21)
  change of local coordinate axis/1 -> Mux/2
  "change of local coordinate axis  "/1 -> Terminator4/1
  Mux/1 -> Linear Displacement 27/1
  MATLAB Function1/10(U2nd) -> Terminator7/1  "Displacement 2nd story"

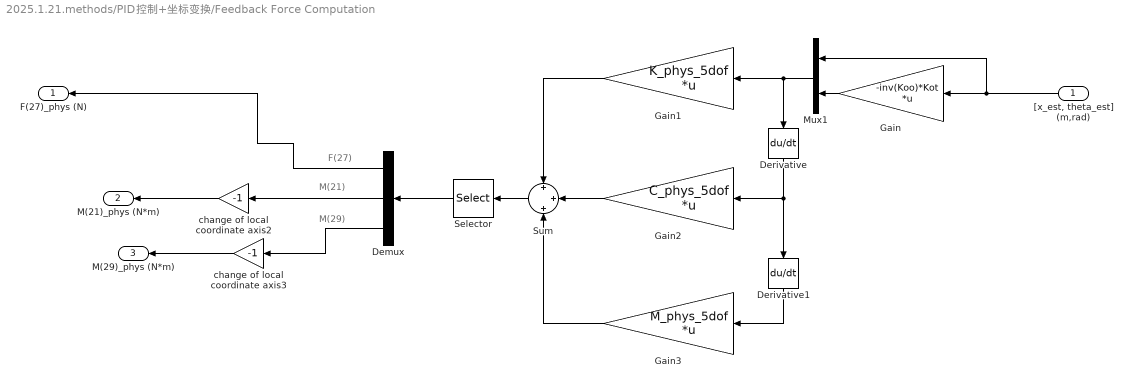
== system 2025.1.21.methods/PID控制+坐标变换/Feedback Force Computation ==
  note: F(27)
  note: M(21)
  note: M(29)
  "[x_est, theta_est] (m,rad)" : Inport
  Demux : Demux  Outputs=3
  Derivative : Derivative
  Derivative1 : Derivative
  Gain : Gain  Gain=-inv(Koo)*Kot  Multiplication=Matrix(K*u) (u vector)
  Gain1 : Gain  Gain=K_phys_5dof  Multiplication=Matrix(K*u) (u vector)
  Gain2 : Gain  Gain=C_phys_5dof  Multiplication=Matrix(K*u) (u vector)
  Gain3 : Gain  Gain=M_phys_5dof  Multiplication=Matrix(K*u) (u vector)
  Mux1 : Mux  Inputs=2
  Selector : Selector  InputPortWidth=5  IndexOptions=Index vector (dialog)  Indices=[1 2 3]  OutputSizes=1
  Sum : Sum  Inputs=+|+|+
  change of local coordinate axis2 : Gain  Gain=-1
  change of local coordinate axis3 : Gain  Gain=-1
  F(27)_phys (N) : Outport  VectorParamsAs1DForOutWhenUnconnected=off
  M(21)_phys (N*m) : Outport  Port=2  VectorParamsAs1DForOutWhenUnconnected=off
  M(29)_phys (N*m) : Outport  Port=3  VectorParamsAs1DForOutWhenUnconnected=off
  wires:
  Gain/1 -> Mux1/2
  Derivative1/1 -> Gain3/1
  Gain2/1 -> Sum/2
  Derivative/1 -> Gain2/1, Derivative1/1
  Gain1/1 -> Sum/1
  "[x_est, theta_est] (m,rad)"/1 -> Gain/1, Mux1/1
  Demux/1 -> F(27)_phys (N)/1
  Sum/1 -> Selector/1
  Selector/1 -> Demux/1
  Gain3/1 -> Sum/3
  Demux/2 -> change of local coordinate axis2/1
  Demux/3 -> change of local coordinate axis3/1
  Mux1/1 -> Derivative/1, Gain1/1
  change of local coordinate axis2/1 -> M(21)_phys (N*m)/1
  change of local coordinate axis3/1 -> M(29)_phys (N*m)/1

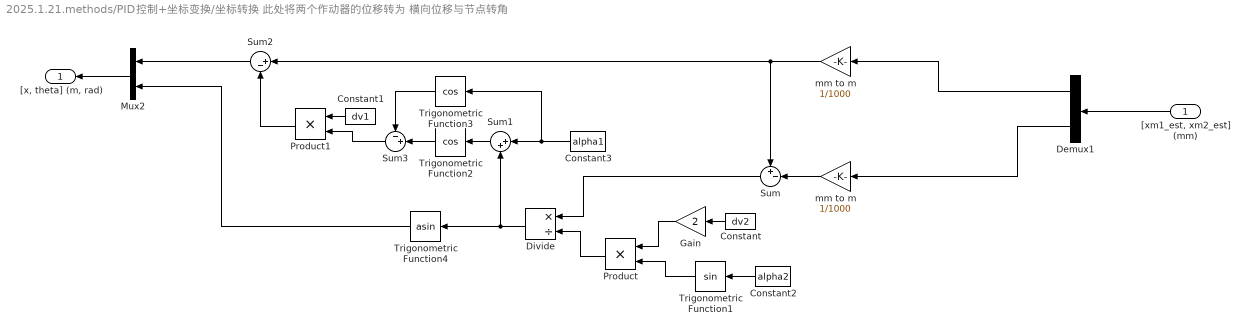
== system 2025.1.21.methods/PID控制+坐标变换/坐标转换 此处将两个作动器的位移转为 横向位移与节点转角  ==
  "[xm1_est, xm2_est] (mm)" : Inport
  Constant : Constant  Value=dv2
  Constant1 : Constant  Value=dv1
  Constant2 : Constant  Value=alpha2
  Constant3 : Constant  Value=alpha1
  Demux1 : Demux  Outputs=2
  Divide : Product  Inputs=*/
  Gain : Gain  Gain=2
  Mux2 : Mux  Inputs=2
  Product : Product
  Product1 : Product
  Sum : Sum  Inputs=+-|
  Sum1 : Sum  Inputs=|++
  Sum2 : Sum  Inputs=|+-
  Sum3 : Sum  Inputs=-+|
  Trigonometric Function1 : Trigonometry
  Trigonometric Function2 : Trigonometry  Operator=cos
  Trigonometric Function3 : Trigonometry  Operator=cos
  Trigonometric Function4 : Trigonometry  Operator=asin
  mm to m : Gain  Gain=1/1000
  "mm to m " : Gain  Gain=1/1000
  "[x, theta] (m, rad)" : Outport  VectorParamsAs1DForOutWhenUnconnected=off
  wires:
  Constant2/1 -> Trigonometric Function1/1
  Constant1/1 -> Product1/1
  Demux1/1 -> mm to m/1
  Demux1/2 -> "mm to m "/1
  Sum/1 -> Divide/1
  Constant/1 -> Gain/1
  Trigonometric Function1/1 -> Product/2
  Gain/1 -> Product/1
  Product/1 -> Divide/2
  Divide/1 -> Sum1/2, Trigonometric Function4/1
  Sum1/1 -> Trigonometric Function2/1
  Constant3/1 -> Sum1/1, Trigonometric Function3/1
  Sum3/1 -> Product1/2
  Sum2/1 -> Mux2/1
  Trigonometric Function2/1 -> Sum3/2
  Trigonometric Function3/1 -> Sum3/1
  Product1/1 -> Sum2/2
  mm to m/1 -> Sum2/1, Sum/1
  "mm to m "/1 -> Sum/2
  Trigonometric Function4/1 -> Mux2/2
  "[xm1_est, xm2_est] (mm)"/1 -> Demux1/1
  Mux2/1 -> "[x, theta] (m, rad)"/1

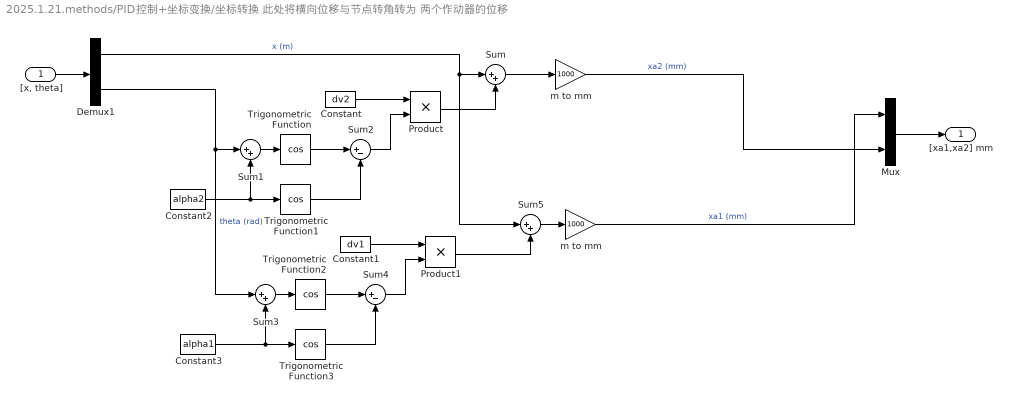
== system 2025.1.21.methods/PID控制+坐标变换/坐标转换 此处将横向位移与节点转角转为 两个作动器的位移 ==
  "[x, theta]" : Inport
  Constant : Constant  Value=dv2
  Constant1 : Constant  Value=dv1
  Constant2 : Constant  Value=alpha2
  Constant3 : Constant  Value=alpha1
  Demux1 : Demux  Outputs=2
  Mux : Mux  Inputs=2
  Product : Product
  Product1 : Product
  Sum{,1,3,5} (4 alike) : Sum  Inputs=|++
  Sum2 : Sum  Inputs=|+-
  Sum4 : Sum  Inputs=|+-
  Trigonometric Function{,1..3} (4 alike) : Trigonometry  Operator=cos
  m to mm : Gain  Gain=1000
  "m to mm " : Gain  Gain=1000
  "[xa1,xa2] mm" : Outport  VectorParamsAs1DForOutWhenUnconnected=off
  wires:
  Constant/1 -> Product/1
  Constant2/1 -> Sum1/2, Trigonometric Function1/1
  Sum1/1 -> Trigonometric Function/1
  Trigonometric Function/1 -> Sum2/1
  Trigonometric Function1/1 -> Sum2/2
  Sum2/1 -> Product/2
  Product/1 -> Sum/2
  Sum/1 -> m to mm/1
  Sum4/1 -> Product1/2
  Trigonometric Function3/1 -> Sum4/2
  Trigonometric Function2/1 -> Sum4/1
  Sum3/1 -> Trigonometric Function2/1
  Constant3/1 -> Sum3/2, Trigonometric Function3/1
  Constant1/1 -> Product1/1
  Product1/1 -> Sum5/2
  Sum5/1 -> "m to mm "/1
  "m to mm "/1 -> Mux/1  "xa1 (mm)"
  m to mm/1 -> Mux/2  "xa2 (mm)"
  Demux1/1 -> Sum/1, Sum5/1  "x (m)"
  "[x, theta]"/1 -> Demux1/1
  Demux1/2 -> Sum3/1, Sum1/1  "theta (rad)"
  Mux/1 -> "[xa1,xa2] mm"/1

== system 2025.1.21.methods/PID控制+坐标变换/控制器与作动器 ==
  Target actuator displacement vector (mm) : Inport
  Control Plant4 : StateSpace  A=A_cplant  B=B_cplant  C=C_cplant  D=D_cplant  InitialCondition=0
  Demux7 : Demux  Outputs=2
  Mux4 : Mux  Inputs=2
  PID Controller2 : slpidlib/PID Controller  Controller=PID  Form=Parallel  TimeDomain=Discrete-time  UseExternalTs=off  SampleTime=-1  IntegratorMethod=Forward Euler  FilterMethod=Forward Euler  ControllerParametersSource=internal  P=1  I=50  UseKiTs=off  D=1e-10  N=100  UseFilter=off  TunerSelectOption=Transfer Function Based (PID Tuner App)  InitialConditionSource=internal  InitialConditionForIntegrator=0  InitialConditionForFilter=0  DifferentiatorICPrevScaledInput=0  ExternalReset=none  TrackingMode=off  Kt=1  LimitOutput=off  SatLimitsSource=internal  UpperSaturationLimit=inf  LowerSaturationLimit=-inf  LinearizeAsGain=on  AntiWindupMode=none  Kb=1  LimitIntegrator=off  UpperIntegratorSaturationLimit=inf  LowerIntegratorSaturationLimit=-inf  POutMin=[]  POutMax=[]  IOutMin=[]  IOutMax=[]  DOutMin=[]  DOutMax=[]  NOutMin=[]  NOutMax=[]  SumOutMin=[]  SumOutMax=[]  SaturationOutMin=[]  SaturationOutMax=[]  PParamMin=[]  PParamMax=[]  IParamMin=[]  IParamMax=[]  DParamMin=[]  DParamMax=[]  NParamMin=[]  NParamMax=[]  KbParamMin=[]  KbParamMax=[]  KtParamMin=[]  KtParamMax=[]  KbOutMin=[]  KbOutMax=[]  KtOutMin=[]  KtOutMax=[]  IntegratorOutMin=[]  IntegratorOutMax=[]  FilterOutMin=[]  FilterOutMax=[]  SumI1OutMin=[]  SumI1OutMax=[]  SumI2OutMin=[]  SumI2OutMax=[]  SumI3OutMin=[]  SumI3OutMax=[]  SumI4OutMin=[]  SumI4OutMax=[]  SumDOutMin=[]  SumDOutMax=[]  DifferentiatorOutMin=[]  DifferentiatorOutMax=[]  FilterDiffOutCoefMin=[]  FilterDiffOutCoefMax=[]  ReciprocalOutMin=[]  ReciprocalOutMax=[]  SumDenOutMin=[]  SumDenOutMax=[]  SumNumOutMin=[]  SumNumOutMax=[]  DivideOutMin=[]  DivideOutMax=[]  UdiffTsProdOutMin=[]  UdiffTsProdOutMax=[]  NTsProdOutMin=[]  NTsProdOutMax=[]  UintegralTsProdOutMin=[]  UintegralTsProdOutMax=[]  UngainTsProdOutMin=[]  UngainTsProdOutMax=[]  ClampingZeroOutDataTypeStr=Inherit: Inherit via back propagation  ClampingZeroOutMin=[]  ClampingZeroOutMax=[]  FilterDenConstantOutDataTypeStr=Inherit: Inherit via back propagation  FilterDenConstantOutMin=[]  FilterDenConstantOutMax=[]  PCopyOutDataTypeStr=Inherit: Inherit via back propagation  PCopyOutMin=[]  PCopyOutMax=[]  NCopyOutDataTypeStr=Inherit: Inherit via back propagation  NCopyOutMin=[]  NCopyOutMax=[]  IntegratorContinuousStateAttributes=''  IntegratorStateMustResolveToSignalObject=off  IntegratorRTWStateStorageClass=Auto  FilterContinuousStateAttributes=''  FilterStateMustResolveToSignalObject=off  FilterRTWStateStorageClass=Auto  ParallelPVariant=InternalParameters  IdealPVariant=Disabled  IVariant=InternalParameters  DVariant=InternalParameters  IntegratorVariant=Discrete  SatVariant=Disabled  AWVariant=Passthrough  PCopyVariant=Disabled  TRVariant=Disabled  FdbkBlocksVariant=Forward  IdealPFdbkVariant=Disabled  SatFdbkVariant=Disabled  DerivativeFilterVariant=Differentiator  NVariant=Passthrough  NCopyVariant=Disabled_SignalSpec  FilterICVariant=InternalICsDifferentiator  IntegratorICVariant=InternalICs  ExternalResetVariant=Disabled  TRSumVariant=Passthrough  SumFdbkVariant=Disabled  SumVariant=Sum_PID  TsampFilterVariant=InternalTs  TsampNgainVariant=Passthrough  TsampIntegralVariant=Disabled_SignalSpec  ExternalSaturationOutDataTypeStr=Inherit: Same as second input
  PID Controller4 : slpidlib/PID Controller  Controller=PID  Form=Parallel  TimeDomain=Discrete-time  UseExternalTs=off  SampleTime=-1  IntegratorMethod=Forward Euler  FilterMethod=Forward Euler  ControllerParametersSource=internal  P=1  I=50  UseKiTs=off  D=1e-10  N=100  UseFilter=on  TunerSelectOption=Transfer Function Based (PID Tuner App)  InitialConditionSource=internal  InitialConditionForIntegrator=0  InitialConditionForFilter=0  DifferentiatorICPrevScaledInput=0  ExternalReset=none  TrackingMode=off  Kt=1  LimitOutput=off  SatLimitsSource=internal  UpperSaturationLimit=inf  LowerSaturationLimit=-inf  LinearizeAsGain=on  AntiWindupMode=none  Kb=1  LimitIntegrator=off  UpperIntegratorSaturationLimit=inf  LowerIntegratorSaturationLimit=-inf  POutMin=[]  POutMax=[]  IOutMin=[]  IOutMax=[]  DOutMin=[]  DOutMax=[]  NOutMin=[]  NOutMax=[]  SumOutMin=[]  SumOutMax=[]  SaturationOutMin=[]  SaturationOutMax=[]  PParamMin=[]  PParamMax=[]  IParamMin=[]  IParamMax=[]  DParamMin=[]  DParamMax=[]  NParamMin=[]  NParamMax=[]  KbParamMin=[]  KbParamMax=[]  KtParamMin=[]  KtParamMax=[]  KbOutMin=[]  KbOutMax=[]  KtOutMin=[]  KtOutMax=[]  IntegratorOutMin=[]  IntegratorOutMax=[]  FilterOutMin=[]  FilterOutMax=[]  SumI1OutMin=[]  SumI1OutMax=[]  SumI2OutMin=[]  SumI2OutMax=[]  SumI3OutMin=[]  SumI3OutMax=[]  SumI4OutMin=[]  SumI4OutMax=[]  SumDOutMin=[]  SumDOutMax=[]  DifferentiatorOutMin=[]  DifferentiatorOutMax=[]  FilterDiffOutCoefMin=[]  FilterDiffOutCoefMax=[]  ReciprocalOutMin=[]  ReciprocalOutMax=[]  SumDenOutMin=[]  SumDenOutMax=[]  SumNumOutMin=[]  SumNumOutMax=[]  DivideOutMin=[]  DivideOutMax=[]  UdiffTsProdOutMin=[]  UdiffTsProdOutMax=[]  NTsProdOutMin=[]  NTsProdOutMax=[]  UintegralTsProdOutMin=[]  UintegralTsProdOutMax=[]  UngainTsProdOutMin=[]  UngainTsProdOutMax=[]  ClampingZeroOutDataTypeStr=Inherit: Inherit via back propagation  ClampingZeroOutMin=[]  ClampingZeroOutMax=[]  FilterDenConstantOutDataTypeStr=Inherit: Inherit via back propagation  FilterDenConstantOutMin=[]  FilterDenConstantOutMax=[]  PCopyOutDataTypeStr=Inherit: Inherit via back propagation  PCopyOutMin=[]  PCopyOutMax=[]  NCopyOutDataTypeStr=Inherit: Inherit via back propagation  NCopyOutMin=[]  NCopyOutMax=[]  IntegratorContinuousStateAttributes=''  IntegratorStateMustResolveToSignalObject=off  IntegratorRTWStateStorageClass=Auto  FilterContinuousStateAttributes=''  FilterStateMustResolveToSignalObject=off  FilterRTWStateStorageClass=Auto  ParallelPVariant=InternalParameters  IdealPVariant=Disabled  IVariant=InternalParameters  DVariant=InternalParameters  IntegratorVariant=Discrete  SatVariant=Disabled  AWVariant=Passthrough  PCopyVariant=Disabled  TRVariant=Disabled  FdbkBlocksVariant=Forward  IdealPFdbkVariant=Disabled  SatFdbkVariant=Disabled  DerivativeFilterVariant=ForwardEulerFilter  NVariant=InternalParameters  NCopyVariant=Disabled  FilterICVariant=InternalICsFilter  IntegratorICVariant=InternalICs  ExternalResetVariant=Disabled  TRSumVariant=Passthrough  SumFdbkVariant=Disabled  SumVariant=Sum_PID  TsampFilterVariant=InternalTs  TsampNgainVariant=Passthrough  TsampIntegralVariant=Disabled_SignalSpec  ExternalSaturationOutDataTypeStr=Inherit: Same as second input
  Sum11 : Sum  Inputs=|+-
  Filtered actuator displacement vector : Outport
  wires:
  PID Controller4/1 -> Mux4/2
  Control Plant4/1 -> Sum11/2, Filtered actuator displacement vector/1  "Filtered actuator displacement vector"
  Demux7/1 -> PID Controller2/1
  Sum11/1 -> Demux7/1
  PID Controller2/1 -> Mux4/1
  Mux4/1 -> Control Plant4/1
  Demux7/2 -> PID Controller4/1
  Target actuator displacement vector (mm)/1 -> Sum11/1

== system 2025.1.21.methods/离散时间下封装模块/Feedback Force Computation2 ==
  "[x_est, theta_est] (m,rad)" : Inport
  Derivative : Derivative
  Derivative1 : Derivative
  Gain1 : Gain  Gain=K_phys_5dof  Multiplication=Matrix(K*u) (u vector)
  Gain2 : Gain  Gain=C_phys_5dof  Multiplication=Matrix(K*u) (u vector)
  Gain3 : Gain  Gain=M_phys_5dof  Multiplication=Matrix(K*u) (u vector)
  Sum : Sum  Inputs=+|+|+
  F(27)_phys (N) : Outport  VectorParamsAs1DForOutWhenUnconnected=off
  wires:
  Derivative1/1 -> Gain3/1
  Gain2/1 -> Sum/2
  Derivative/1 -> Gain2/1, Derivative1/1
  Gain1/1 -> Sum/1
  Sum/1 -> F(27)_phys (N)/1
  Gain3/1 -> Sum/3
  "[x_est, theta_est] (m,rad)"/1 -> Derivative/1, Gain1/1

== system 2025.1.21.methods/连续时间下封装模块/Feedback Force Computation1 ==
  "[x_est, theta_est] (m,rad)" : Inport
  Derivative : Derivative
  Derivative1 : Derivative
  Gain1 : Gain  Gain=K_phys_5dof  Multiplication=Matrix(K*u) (u vector)
  Gain2 : Gain  Gain=C_phys_5dof  Multiplication=Matrix(K*u) (u vector)
  Gain3 : Gain  Gain=M_phys_5dof  Multiplication=Matrix(K*u) (u vector)
  Sum : Sum  Inputs=+|+|+
  F(27)_phys (N) : Outport  VectorParamsAs1DForOutWhenUnconnected=off
  wires:
  Derivative1/1 -> Gain3/1
  Gain2/1 -> Sum/2
  Derivative/1 -> Gain2/1, Derivative1/1
  Gain1/1 -> Sum/1
  Sum/1 -> F(27)_phys (N)/1
  Gain3/1 -> Sum/3
  "[x_est, theta_est] (m,rad)"/1 -> Derivative/1, Gain1/1

== matlab function 2025.1.21.methods/LQG+坐标变换/ NUMERICAL SUBSTRUCTURE/MATLAB Function1 ==
  data: U27_MA output; V27_MA output; A27_MA output; Theta21_MA output; VTheta21_MA output; ATheta21_MA output; Theta29_MA output; VTheta29_MA output; ATheta29_MA output; U2nd output; Theta2nd output; U3rd output; Theta3rd output; U1 output; Vel1 output; Acc1 output; accel_grd input; FB_force27 input; FB_moment29 input; FB_moment21 input; Kbar_inv input; MNrt input; CNrt input; Ag input; l input; Rbar input; F input; U0 input; Vel0 input; Acc0 input; a0 parameter; a1 parameter; a2 parameter; a3 parameter; a4 parameter; a5 parameter; a6 parameter; a7 parameter
function [U27_MA,V27_MA,A27_MA,Theta21_MA,VTheta21_MA,ATheta21_MA,Theta29_MA,VTheta29_MA,ATheta29_MA,U2nd,Theta2nd,U3rd,Theta3rd,U1,Vel1,Acc1]=...
    fcn(accel_grd,FB_force27,FB_moment29,FB_moment21,Kbar_inv, MNrt, CNrt,Ag,l,Rbar,F,...
    U0,Vel0,Acc0, a0, a1, a2, a3, a4, a5, a6, a7)
             
             
    % ============================
	% *  Update next iteration   *
	% ============================
    ndof = length(Kbar_inv);
    U1   = zeros(ndof,1);
    Vel1 = zeros(ndof,1);
    Acc1 = zeros(ndof,1);
    
    U27_MA = 0;
    V27_MA = 0;
    A27_MA = 0;

    Theta21_MA = 0;
    VTheta21_MA = 0;
    ATheta21_MA = 0;
% 
%     U6_MA = 0;
%     V6_MA = 0;
%     A6_MA = 0;
    U2nd = 0 ;              %Displacement 2nd story, node 12, DOF 26
    Theta2nd = 0;          %Rotation 2nd story, node 12, DOF 22
    U3rd = 0;              %Displacement 3rd story, node 16, DOF 13
    Theta3rd = 0;           %Rotation 3rd story, node 16, DOF 3


    Theta29_MA = 0;
    VTheta29_MA = 0;
    ATheta29_MA = 0;

    % ============================
	% *  Feedback Force / Moment *
	% ============================
    F(27) = FB_force27;
    F(21) = FB_moment21;
    F(29) = FB_moment29;

    % ==========================
	% *     Update Matrices    *
	% ==========================
    Ag(:)  = accel_grd * l;
    
   	% ==========================
	% * 	  Form Rbar  	   *
	% ==========================
	Rbar = ( (MNrt * ((a0*U0)+(a2*Vel0)+(a3*Acc0))) + ...
		     (CNrt * ((a1*U0)+(a4*Vel0)+(a5*Acc0))) - F - (MNrt * Ag) );
    
    % ==========================
	% * Solve for Displacement *
	% ==========================
	U1 = Kbar_inv * Rbar;
    
	% ============================
	% * Compute Velocity & Accel *
	% ============================
	Acc1=a0*(U1-U0)-a2*Vel0-a3*Acc0;
	Vel1=Vel0+a7*Acc1+a6*Acc0; 

	% ============================
	% *    Output u1 and theta   *
	% ============================
    U27_MA    = U1(27);
    V27_MA    = Vel1(27);
    A27_MA    = Acc1(27);    

%     U6_MA    = U1(27);
%     V6_MA    = Vel1(27);
%     A6_MA    = Acc1(27);

    Theta21_MA = U1(21);
    VTheta21_MA = Vel1(21);
    ATheta21_MA = Acc1(21);

    Theta29_MA = U1(29);
    VTheta29_MA = Vel1(29);
    ATheta29_MA = Acc1(29);
    
    % ADDED by Johnny
    U2nd = U1(26);              %Displacement 2nd story, node 12, DOF 26
    Theta2nd = U1(22);          %Rotation 2nd story, node 12, DOF 22
    U3rd = U1(13);              %Displacement 3rd story, node 16, DOF 13
    Theta3rd = U1(3);           %Rotation 3rd story, node 16, DOF 3

end

== matlab function 2025.1.21.methods/PID控制+坐标变换/ 数值子结构/MATLAB Function1 ==
  data: U27_MA output; V27_MA output; A27_MA output; Theta21_MA output; VTheta21_MA output; ATheta21_MA output; Theta29_MA output; VTheta29_MA output; ATheta29_MA output; U2nd output; Theta2nd output; U3rd output; Theta3rd output; U1 output; Vel1 output; Acc1 output; accel_grd input; FB_force27 input; FB_moment29 input; FB_moment21 input; Kbar_inv input; MNrt input; CNrt input; Ag input; l input; Rbar input; F input; U0 input; Vel0 input; Acc0 input; a0 parameter; a1 parameter; a2 parameter; a3 parameter; a4 parameter; a5 parameter; a6 parameter; a7 parameter
function [U27_MA,V27_MA,A27_MA,Theta21_MA,VTheta21_MA,ATheta21_MA,Theta29_MA,VTheta29_MA,ATheta29_MA,U2nd,Theta2nd,U3rd,Theta3rd,U1,Vel1,Acc1]=...
    fcn(accel_grd,FB_force27,FB_moment29,FB_moment21,Kbar_inv, MNrt, CNrt,Ag,l,Rbar,F,...
    U0,Vel0,Acc0, a0, a1, a2, a3, a4, a5, a6, a7)
             
             
    % ============================
	% *  Update next iteration   *
	% ============================
    ndof = length(Kbar_inv);
    U1   = zeros(ndof,1);
    Vel1 = zeros(ndof,1);
    Acc1 = zeros(ndof,1);
    
    U27_MA = 0;
    V27_MA = 0;
    A27_MA = 0;

    Theta21_MA = 0;
    VTheta21_MA = 0;
    ATheta21_MA = 0;
% 
%     U6_MA = 0;
%     V6_MA = 0;
%     A6_MA = 0;
    U2nd = 0 ;              %Displacement 2nd story, node 12, DOF 26
    Theta2nd = 0;          %Rotation 2nd story, node 12, DOF 22
    U3rd = 0;              %Displacement 3rd story, node 16, DOF 13
    Theta3rd = 0;           %Rotation 3rd story, node 16, DOF 3


    Theta29_MA = 0;
    VTheta29_MA = 0;
    ATheta29_MA = 0;

    % ============================
	% *  Feedback Force / Moment *
	% ============================
    F(27) = FB_force27;
    F(21) = FB_moment21;
    F(29) = FB_moment29;

    % ==========================
	% *     Update Matrices    *
	% ==========================
    Ag(:)  = accel_grd * l;
    
   	% ==========================
	% * 	  Form Rbar  	   *
	% ==========================
	Rbar = ( (MNrt * ((a0*U0)+(a2*Vel0)+(a3*Acc0))) + ...
		     (CNrt * ((a1*U0)+(a4*Vel0)+(a5*Acc0))) - F - (MNrt * Ag) );
    
    % ==========================
	% * Solve for Displacement *
	% ==========================
	U1 = Kbar_inv * Rbar;
    
	% ============================
	% * Compute Velocity & Accel *
	% ============================
	Acc1=a0*(U1-U0)-a2*Vel0-a3*Acc0;
	Vel1=Vel0+a7*Acc1+a6*Acc0; 

	% ============================
	% *    Output u1 and theta   *
	% ============================
    U27_MA    = U1(27);
    V27_MA    = Vel1(27);
    A27_MA    = Acc1(27);    

%     U6_MA    = U1(27);
%     V6_MA    = Vel1(27);
%     A6_MA    = Acc1(27);

    Theta21_MA = U1(21);
    VTheta21_MA = Vel1(21);
    ATheta21_MA = Acc1(21);

    Theta29_MA = U1(29);
    VTheta29_MA = Vel1(29);
    ATheta29_MA = Acc1(29);
    
    % ADDED by Johnny
    U2nd = U1(26);              %Displacement 2nd story, node 12, DOF 26
    Theta2nd = U1(22);          %Rotation 2nd story, node 12, DOF 22
    U3rd = U1(13);              %Displacement 3rd story, node 16, DOF 13
    Theta3rd = U1(3);           %Rotation 3rd story, node 16, DOF 3

end
